simulink model "winter_simulink_2019"  (R2022a)
settings: Solver=FixedStepAuto  StartTime=0  StopTime=stop_time  FixedStep=simulation.time_step  RelTol=1e-3
values from neighbouring files (symbols this model uses):
  I_eq = param{1}    [main_IMM.m]    (also in parameters_old.m = rotor.I + generator.I/gearbox.ratio^2)
  lambda_vector = linspace(lambda_range(1), lambda_range(2), lambda_item)    [parameters_old.m]
  omega_rated = rated_values(2)    [parameters_old.m]
  pitch_range = deg2rad([-15 90])    [parameters_old.m]
  pitch_vector = linspace(pitch_range(1), pitch_range(2), pitch_item)    [parameters_old.m]
  rho = param{2}    [main_IMM.m]    (also in parameters_old.m = 1.225)
undefined symbols (not defined in the file or in its folder): blade, Gc, gearbox, generator, lookup_cP, omega_r, Riq, rotor, wind, Yiq
settings Model: Creator=Niccolò  LastModifiedBy=Niccolò
settings SolverCC: AlgebraicLoopSolver=TrustRegion

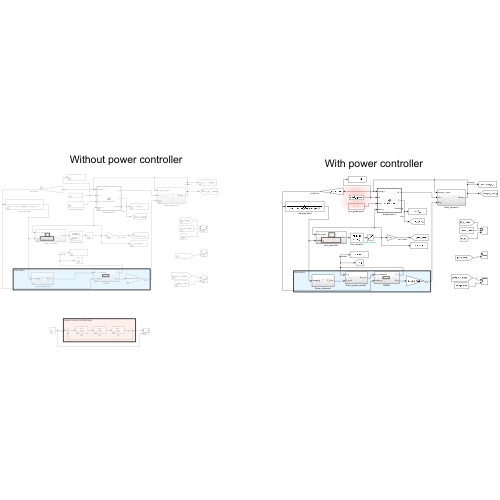
[thumbnail: Simulink's stored preview of the top-level diagram]
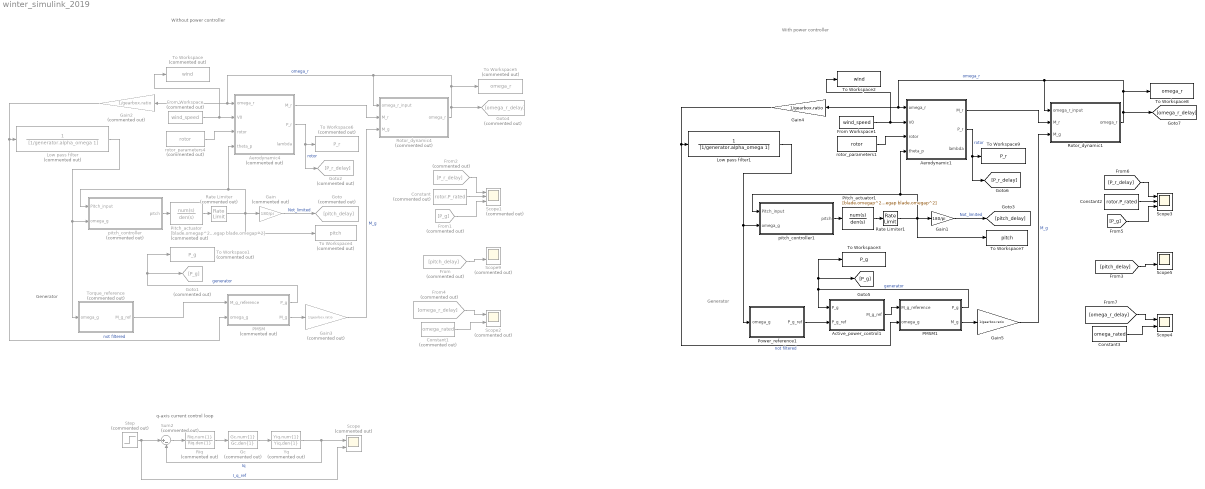
== system winter_simulink_2019 ==
  note: Without power controller
  note: Generator
  note: q-axis current control loop
  note: Generator
  note: With power controller
  Active_power_control1 : Subsystem
  Aerodynamic1 : MATLAB Function  TreatAsAtomicUnit=on
  Aerodynamic4 : MATLAB Function  Commented=on  TreatAsAtomicUnit=on
  Constant : Constant  Commented=on  Value=rotor.P_rated
  Constant1 : Constant  Commented=on  Value=omega_rated
  Constant2 : Constant  Value=rotor.P_rated
  Constant3 : Constant  Value=omega_rated
  From : From  Commented=on  GotoTag=pitch_delay
  From Workspace : FromWorkspace  Commented=on  VariableName=wind_speed  SampleTime=1/wind.sample_f
  From Workspace1 : FromWorkspace  VariableName=wind_speed  SampleTime=1/wind.sample_f
  From1 : From  Commented=on  GotoTag=P_g
  From2 : From  Commented=on  GotoTag=P_r_delay
  From4 : From  Commented=on  GotoTag=omega_r_delay
  Gain : Gain  Commented=on  Gain=180/pi
  Gain1 : Gain  Gain=180/pi
  Gain2 : Gain  Commented=on  Gain=1/gearbox.ratio
  Gain3 : Gain  Commented=on  Gain=1/gearbox.ratio
  Gain4 : Gain  Gain=1/gearbox.ratio
  Gain5 : Gain  Gain=1/gearbox.ratio
  Gc : TransferFcn  Commented=on  Numerator=Gc.num{1}  Denominator=Gc.den{1}
  Goto : Goto  Commented=on  GotoTag=pitch_delay
  Goto1 : Goto  Commented=on  GotoTag=P_g
  Goto2 : Goto  Commented=on  GotoTag=P_r_delay
  Goto4 : Goto  Commented=on  GotoTag=omega_r_delay
  Low pass filter : TransferFcn  Commented=on  Denominator=[1/generator.alpha_omega 1]
  Low pass filter1 : TransferFcn  Denominator=[1/generator.alpha_omega 1]
  PMSM : Subsystem  Commented=on
  PMSM1 : Subsystem
  Pitch_actuator : TransferFcn  Commented=on  Numerator=[blade.omegap^2]  Denominator=[1 2*blade.zetap*blade.omegap blade.omegap^2]
  Pitch_actuator1 : TransferFcn  Numerator=[blade.omegap^2]  Denominator=[1 2*blade.zetap*blade.omegap blade.omegap^2]
  Power_reference1 : Subsystem
  Rate Limiter : RateLimiter  Commented=on  RisingSlewLimit=blade.pitch_rate  FallingSlewLimit=-blade.pitch_rate  SampleTimeMode=inherited
  Rate Limiter1 : RateLimiter  RisingSlewLimit=blade.pitch_rate  FallingSlewLimit=-blade.pitch_rate  SampleTimeMode=inherited
  Riq : TransferFcn  Commented=on  Numerator=Riq.num{1}  Denominator=Riq.den{1}
  Rotor_dynamic1 : Subsystem
  Rotor_dynamic4 : Subsystem  Commented=on
  Scope : Scope  Commented=on  NumInputPorts=2
  Scope1 : Scope  Commented=on  NumInputPorts=3
  Scope2 : Scope  Commented=on  NumInputPorts=2
  Scope3 : Scope  NumInputPorts=3
  Scope4 : Scope  NumInputPorts=2
  Scope5 : Scope  NumInputPorts=2
  Scope9 : Scope  Commented=on  NumInputPorts=2
  Step : Step  Commented=on  SampleTime=0
  Sum2 : Sum  Commented=on  Inputs=|+-
  To Workspace : ToWorkspace  Commented=on  VariableName=wind  SaveFormat=Timeseries  SampleTime=-1
  To Workspace1 : ToWorkspace  Commented=on  VariableName=P_g  SaveFormat=Timeseries  SampleTime=-1
  To Workspace2 : ToWorkspace  VariableName=wind  SaveFormat=Timeseries  SampleTime=-1
  To Workspace3 : ToWorkspace  VariableName=P_g  SaveFormat=Timeseries  SampleTime=-1
  To Workspace4 : ToWorkspace  Commented=on  VariableName=pitch  SaveFormat=Timeseries  SampleTime=-1
  To Workspace5 : ToWorkspace  Commented=on  VariableName=omega_r  SaveFormat=Timeseries  SampleTime=-1
  To Workspace6 : ToWorkspace  Commented=on  VariableName=P_r  SaveFormat=Timeseries  SampleTime=-1
  To Workspace7 : ToWorkspace  VariableName=pitch  SaveFormat=Timeseries  SampleTime=-1
  To Workspace8 : ToWorkspace  VariableName=omega_r  SaveFormat=Timeseries  SampleTime=-1
  To Workspace9 : ToWorkspace  VariableName=P_r  SaveFormat=Timeseries  SampleTime=-1
  Torque_reference : Subsystem  Commented=on
  Yq : TransferFcn  Commented=on  Numerator=Yiq.num{1}  Denominator=Yiq.den{1}
  pitch_controller : Subsystem  Commented=on
  pitch_controller1 : Subsystem
  rotor_parameters1 : Constant  Value=rotor  OutDataTypeStr=Bus: rotor_bus
  rotor_parameters4 : Constant  Commented=on  Value=rotor  OutDataTypeStr=Bus: rotor_bus
  wires:
  Aerodynamic4/1(M_r) -> Rotor_dynamic4/2(M_r)
  From Workspace/1 -> To Workspace/1, Aerodynamic4/2(V0)
  rotor_parameters4/1 -> Aerodynamic4/3(rotor)
  Gain2/1 -> PMSM/2(omega_g), Low pass filter/1  "not filtered"
  Rotor_dynamic4/1(omega_r) -> Goto4/1, Gain2/1, Aerodynamic4/1(omega_r), Rotor_dynamic4/1(omega_r_input), To Workspace5/1  "omega_r"
  Aerodynamic4/2(P_r) -> Goto2/1, To Workspace6/1  "rotor"
  Gain/1 -> Goto/1  "Not_limited"
  PMSM/1(P_g) -> To Workspace1/1, Goto1/1  "generator"
  pitch_controller/1(pitch) -> Pitch_actuator/1
  PMSM/2(M_g) -> Gain3/1
  Gain3/1 -> Rotor_dynamic4/3(M_g)  "M_g"
  Step/1 -> Scope/2, Sum2/1  "I_q_ref"
  Gc/1 -> Yq/1
  Riq/1 -> Gc/1
  Yq/1 -> Scope/1, Sum2/2  "Iq"
  Sum2/1 -> Riq/1
  Low pass filter/1 -> Torque_reference/1(omega_g), pitch_controller/2(omega_g)
  Pitch_actuator/1 -> Rate Limiter/1
  Rate Limiter/1 -> Aerodynamic4/4(theta_p), pitch_controller/1(Pitch_input), Gain/1, To Workspace4/1
  From/1 -> Scope9/2
  From2/1 -> Scope1/1
  Constant/1 -> Scope1/2
  From4/1 -> Scope2/1
  From1/1 -> Scope1/3
  Constant1/1 -> Scope2/2
  Torque_reference/1(M_g_ref) -> PMSM/1(M_g_reference)
  From Workspace1/1 -> To Workspace2/1, Aerodynamic1/2(V0)
  Aerodynamic1/2(P_r) -> [P_r_delay], To Workspace9/1  "rotor"
  [pitch_delay] -> Scope5/2
  Gain4/1 -> PMSM1/2(omega_g), Low pass filter1/1  "not filtered"
  Rate Limiter1/1 -> Aerodynamic1/4(theta_p), pitch_controller1/1(Pitch_input), Gain1/1, To Workspace7/1
  pitch_controller1/1(pitch) -> Pitch_actuator1/1
  [P_r_delay] -> Scope3/1
  Constant3/1 -> Scope4/2
  Constant2/1 -> Scope3/2
  [omega_r_delay] -> Scope4/1
  Low pass filter1/1 -> Power_reference1/1(omega_g), pitch_controller1/2(omega_g)
  Gain1/1 -> [pitch_delay]  "Not_limited"
  Gain5/1 -> Rotor_dynamic1/3(M_g)  "M_g"
  PMSM1/2(M_g) -> Gain5/1
  Aerodynamic1/1(M_r) -> Rotor_dynamic1/2(M_r)
  [P_g] -> Scope3/3
  rotor_parameters1/1 -> Aerodynamic1/3(rotor)
  PMSM1/1(P_g) -> Active_power_control1/1(P_g), To Workspace3/1, [P_g]  "generator"
  Pitch_actuator1/1 -> Rate Limiter1/1
  Power_reference1/1(P_g_ref) -> Active_power_control1/2(P_g_ref)
  Active_power_control1/1(M_g_ref) -> PMSM1/1(M_g_reference)
  Rotor_dynamic1/1(omega_r) -> [omega_r_delay], Gain4/1, Aerodynamic1/1(omega_r), Rotor_dynamic1/1(omega_r_input), To Workspace8/1  "omega_r"

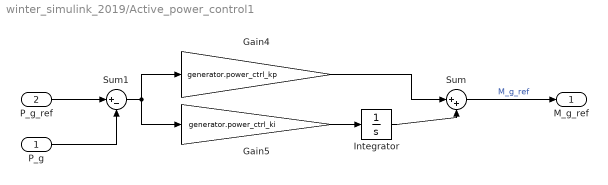
== system winter_simulink_2019/Active_power_control1 ==
  P_g : Inport
  P_g_ref : Inport  Port=2
  Gain4 : Gain  Gain=generator.power_ctrl_kp
  Gain5 : Gain  Gain=generator.power_ctrl_ki
  Integrator : Integrator
  Sum : Sum  Inputs=|++
  Sum1 : Sum  Inputs=|+-
  M_g_ref : Outport
  wires:
  P_g/1 -> Sum1/2
  Gain5/1 -> Integrator/1
  Sum1/1 -> Gain4/1, Gain5/1
  Sum/1 -> M_g_ref/1  "M_g_ref"
  Gain4/1 -> Sum/1
  Integrator/1 -> Sum/2
  P_g_ref/1 -> Sum1/1

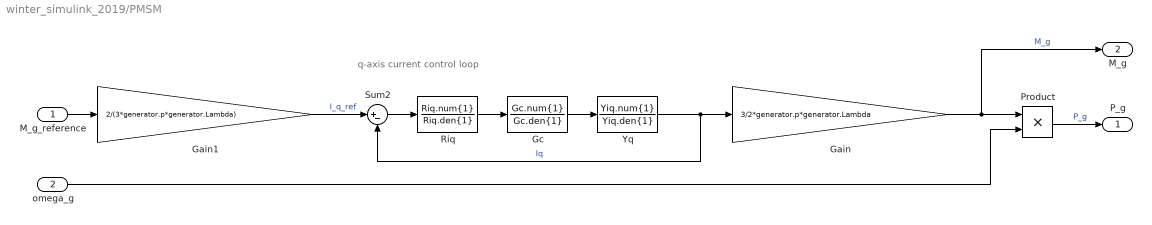
== system winter_simulink_2019/PMSM ==
  note: q-axis current control loop
  M_g_reference : Inport
  omega_g : Inport  Port=2
  Gain : Gain  Gain=3/2*generator.p*generator.Lambda
  Gain1 : Gain  Gain=2/(3*generator.p*generator.Lambda)
  Gc : TransferFcn  Numerator=Gc.num{1}  Denominator=Gc.den{1}
  Product : Product
  Riq : TransferFcn  Numerator=Riq.num{1}  Denominator=Riq.den{1}
  Sum2 : Sum  Inputs=|+-
  Yq : TransferFcn  Numerator=Yiq.num{1}  Denominator=Yiq.den{1}
  P_g : Outport
  M_g : Outport  Port=2
  wires:
  Gc/1 -> Yq/1
  M_g_reference/1 -> Gain1/1
  Gain/1 -> M_g/1, Product/1  "M_g"
  Riq/1 -> Gc/1
  Sum2/1 -> Riq/1
  Yq/1 -> Gain/1, Sum2/2  "Iq"
  Product/1 -> P_g/1  "P_g"
  omega_g/1 -> Product/2
  Gain1/1 -> Sum2/1  "I_q_ref"

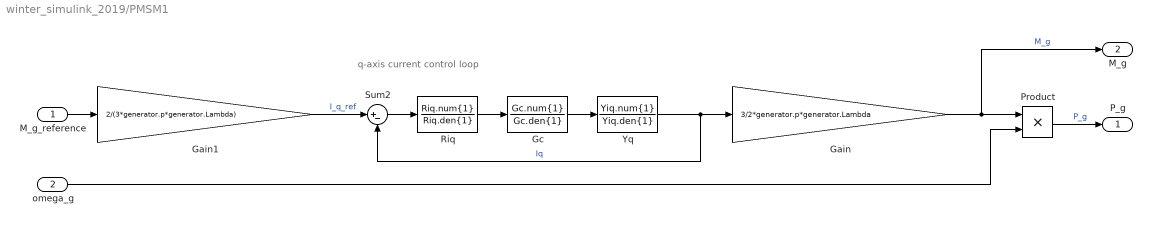
== system winter_simulink_2019/PMSM1 ==
  note: q-axis current control loop
  M_g_reference : Inport
  omega_g : Inport  Port=2
  Gain : Gain  Gain=3/2*generator.p*generator.Lambda
  Gain1 : Gain  Gain=2/(3*generator.p*generator.Lambda)
  Gc : TransferFcn  Numerator=Gc.num{1}  Denominator=Gc.den{1}
  Product : Product
  Riq : TransferFcn  Numerator=Riq.num{1}  Denominator=Riq.den{1}
  Sum2 : Sum  Inputs=|+-
  Yq : TransferFcn  Numerator=Yiq.num{1}  Denominator=Yiq.den{1}
  P_g : Outport
  M_g : Outport  Port=2
  wires:
  Gc/1 -> Yq/1
  M_g_reference/1 -> Gain1/1
  Gain/1 -> M_g/1, Product/1  "M_g"
  Riq/1 -> Gc/1
  Sum2/1 -> Riq/1
  Yq/1 -> Gain/1, Sum2/2  "Iq"
  Product/1 -> P_g/1  "P_g"
  omega_g/1 -> Product/2
  Gain1/1 -> Sum2/1  "I_q_ref"

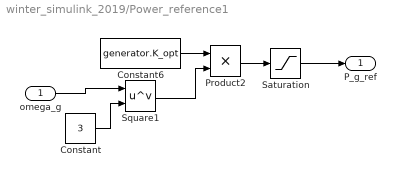
== system winter_simulink_2019/Power_reference1 ==
  omega_g : Inport
  Constant : Constant  Value=3
  Constant6 : Constant  Value=generator.K_opt
  Product2 : Product
  Saturation : Saturate  UpperLimit=rotor.P_rated  LowerLimit=0
  Square1 : Math  Operator=pow
  P_g_ref : Outport
  wires:
  Product2/1 -> Saturation/1
  omega_g/1 -> Square1/1
  Square1/1 -> Product2/2
  Constant6/1 -> Product2/1
  Saturation/1 -> P_g_ref/1
  Constant/1 -> Square1/2

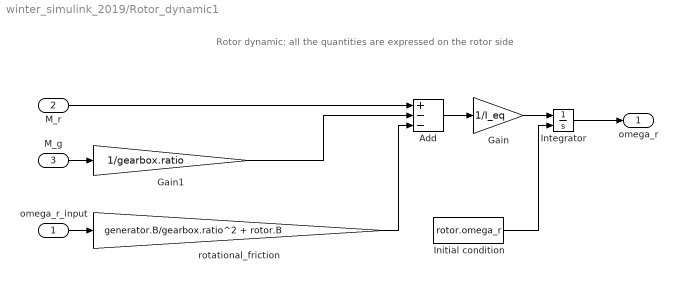
== system winter_simulink_2019/Rotor_dynamic1 ==
  note: Rotor dynamic: all the quantities are expressed on the rotor side
  omega_r_input : Inport
  M_r : Inport  Port=2
  M_g : Inport  Port=3
  Add : Sum  Inputs=+--
  Gain : Gain  Gain=1/I_eq
  Gain1 : Gain  Gain=1/gearbox.ratio
  Initial condition : Constant  Value=rotor.omega_r
  Integrator : Integrator  InitialConditionSource=external  InitialCondition=omega_r
  rotational_friction : Gain  Gain=generator.B/gearbox.ratio^2 + rotor.B
  omega_r : Outport
  wires:
  Add/1 -> Gain/1
  Gain/1 -> Integrator/1
  M_r/1 -> Add/1
  Initial condition/1 -> Integrator/2
  omega_r_input/1 -> rotational_friction/1
  rotational_friction/1 -> Add/3
  M_g/1 -> Gain1/1
  Gain1/1 -> Add/2
  Integrator/1 -> omega_r/1

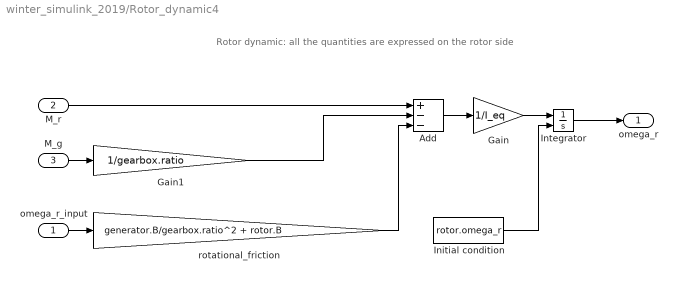
== system winter_simulink_2019/Rotor_dynamic4 ==
  note: Rotor dynamic: all the quantities are expressed on the rotor side
  omega_r_input : Inport
  M_r : Inport  Port=2
  M_g : Inport  Port=3
  Add : Sum  Inputs=+--
  Gain : Gain  Gain=1/I_eq
  Gain1 : Gain  Gain=1/gearbox.ratio
  Initial condition : Constant  Value=rotor.omega_r
  Integrator : Integrator  InitialConditionSource=external  InitialCondition=omega_r
  rotational_friction : Gain  Gain=generator.B/gearbox.ratio^2 + rotor.B
  omega_r : Outport
  wires:
  Add/1 -> Gain/1
  Gain/1 -> Integrator/1
  M_r/1 -> Add/1
  Initial condition/1 -> Integrator/2
  omega_r_input/1 -> rotational_friction/1
  rotational_friction/1 -> Add/3
  M_g/1 -> Gain1/1
  Gain1/1 -> Add/2
  Integrator/1 -> omega_r/1

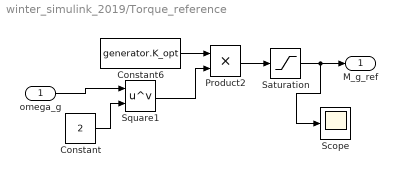
== system winter_simulink_2019/Torque_reference ==
  omega_g : Inport
  Constant : Constant  Value=2
  Constant6 : Constant  Value=generator.K_opt
  Product2 : Product
  Saturation : Saturate  UpperLimit=rotor.P_rated*gearbox.ratio/omega_rated  LowerLimit=0
  Scope : Scope
  Square1 : Math  Operator=pow
  M_g_ref : Outport
  wires:
  Product2/1 -> Saturation/1
  omega_g/1 -> Square1/1
  Square1/1 -> Product2/2
  Constant6/1 -> Product2/1
  Saturation/1 -> Scope/1, M_g_ref/1
  Constant/1 -> Square1/2

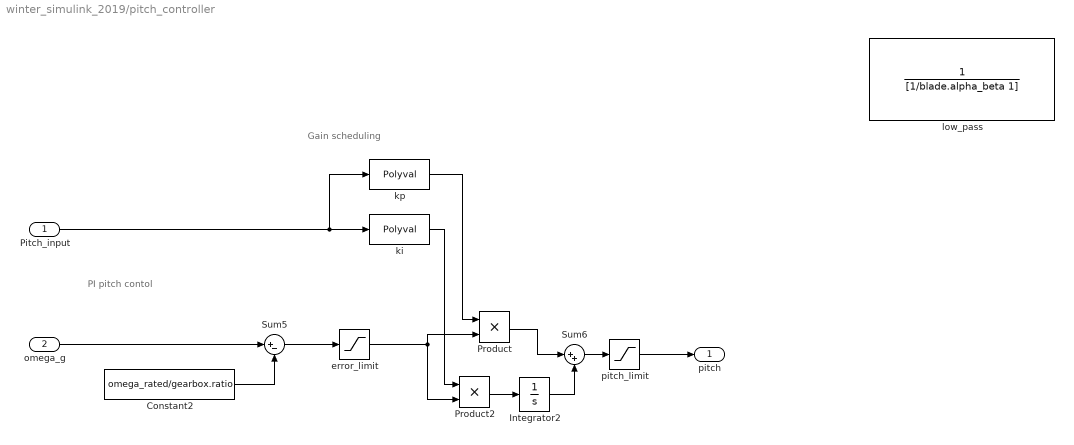
== system winter_simulink_2019/pitch_controller ==
  note: Gain scheduling
  note: PI pitch contol
  Pitch_input : Inport
  omega_g : Inport  Port=2
  Constant2 : Constant  Value=omega_rated/gearbox.ratio
  Integrator2 : Integrator
  Product : Product
  Product2 : Product
  Sum5 : Sum  Inputs=|+-
  Sum6 : Sum  Inputs=|++
  error_limit : Saturate  UpperLimit=10  LowerLimit=-0.15
  ki : Polyval  Coefs=blade.ki_schedule
  kp : Polyval  Coefs=blade.kp_schedule
  low_pass : TransferFcn  Denominator=[1/blade.alpha_beta 1]
  pitch_limit : Saturate  UpperLimit=pitch_range(2)  LowerLimit=0
  pitch : Outport
  wires:
  Sum6/1 -> pitch_limit/1
  omega_g/1 -> Sum5/1
  Product/1 -> Sum6/1
  Constant2/1 -> Sum5/2
  ki/1 -> Product2/1
  kp/1 -> Product/1
  Pitch_input/1 -> kp/1, ki/1
  error_limit/1 -> Product2/2, Product/2
  Integrator2/1 -> Sum6/2
  Product2/1 -> Integrator2/1
  Sum5/1 -> error_limit/1
  pitch_limit/1 -> pitch/1

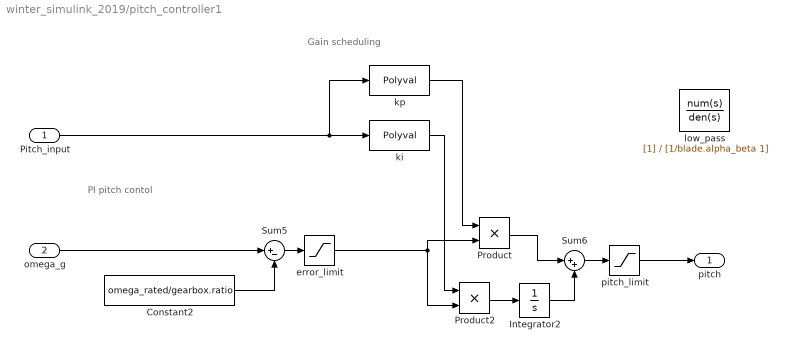
== system winter_simulink_2019/pitch_controller1 ==
  note: Gain scheduling
  note: PI pitch contol
  Pitch_input : Inport
  omega_g : Inport  Port=2
  Constant2 : Constant  Value=omega_rated/gearbox.ratio
  Integrator2 : Integrator
  Product : Product
  Product2 : Product
  Sum5 : Sum  Inputs=|+-
  Sum6 : Sum  Inputs=|++
  error_limit : Saturate  UpperLimit=10  LowerLimit=-0.15
  ki : Polyval  Coefs=blade.ki_schedule
  kp : Polyval  Coefs=blade.kp_schedule
  low_pass : TransferFcn  Denominator=[1/blade.alpha_beta 1]
  pitch_limit : Saturate  UpperLimit=pitch_range(2)  LowerLimit=0
  pitch : Outport
  wires:
  Sum6/1 -> pitch_limit/1
  omega_g/1 -> Sum5/1
  Product/1 -> Sum6/1
  Constant2/1 -> Sum5/2
  ki/1 -> Product2/1
  kp/1 -> Product/1
  Pitch_input/1 -> kp/1, ki/1
  error_limit/1 -> Product2/2, Product/2
  Integrator2/1 -> Sum6/2
  Product2/1 -> Integrator2/1
  Sum5/1 -> error_limit/1
  pitch_limit/1 -> pitch/1

== matlab function winter_simulink_2019/Aerodynamic4 ==
  data: omega_r input; V0 input; M_r output; P_r output; rho parameter; rotor input; theta_p input; lambda_vector parameter; pitch_vector parameter; lookup_cP parameter; lambda output
function [M_r, P_r, lambda] = Aerodynamic(omega_r, V0, rho, rotor, ...
  theta_p, lambda_vector, pitch_vector, lookup_cP) 

R = rotor.R;                  % rotor radius [m]

% retrive the cP from the look-up table
lambda = omega_r*R/V0;                                                
cP = interp2(lambda_vector, pitch_vector, lookup_cP, lambda, theta_p);

P_r = 0.5*rho*V0^3*pi*R^2*cP; % rotor power [W]
M_r = P_r/omega_r;            % rotor torque [Nm]

== matlab function winter_simulink_2019/Aerodynamic1 ==
  data: omega_r input; V0 input; M_r output; P_r output; rho parameter; rotor input; theta_p input; lambda_vector parameter; pitch_vector parameter; lookup_cP parameter; lambda output
function [M_r, P_r, lambda] = Aerodynamic(omega_r, V0, rho, rotor, ...
  theta_p, lambda_vector, pitch_vector, lookup_cP) 

R = rotor.R;                  % rotor radius [m]

% retrive the cP from the look-up table
lambda = omega_r*R/V0;                                                
cP = interp2(lambda_vector, pitch_vector, lookup_cP, lambda, theta_p);

P_r = 0.5*rho*V0^3*pi*R^2*cP; % rotor power [W]
M_r = P_r/omega_r;            % rotor torque [Nm]
